simulink model "buck_boost_sim"  (R2020a)
settings: Solver=FixedStepAuto  StartTime=0.0  StopTime=sim_duration  FixedStep=1e-3  RelTol=1e-3
values from neighbouring files (symbols this model uses):
  A = double(eval(subs(A, u, ue)))    [linearizacija_simbolicki_script.m]    (also in linearizacija_simbolicki_skripta.m)
  B = double(eval(subs(B, [x1, x2], [x1e, x2e])))    [linearizacija_simbolicki_script.m]    (also in linearizacija_simbolicki_skripta.m)
  C = 470e-6    (= 0.00047)    [linearizacija_simbolicki_script.m]    (also in linearizacija_simbolicki_skripta.m)
  E = 12    [linearizacija_simbolicki_script.m]    (also in linearizacija_simbolicki_skripta.m)
  H = [0 1]    [linearizacija_simbolicki_script.m]    (also in linearizacija_simbolicki_skripta.m)
  L = 15.91e-3    (= 0.01591)    [linearizacija_simbolicki_script.m]    (also in linearizacija_simbolicki_skripta.m)
  R = 52    [linearizacija_simbolicki_script.m]    (also in linearizacija_simbolicki_skripta.m)
  sim_duration = 5    [projektovanje_kontrolera_script.m]
  ue = eval(ue)    [linearizacija_simbolicki_script.m]    (also in linearizacija_simbolicki_skripta.m)
  x2e = -22.5    [linearizacija_simbolicki_script.m]    (also in linearizacija_simbolicki_skripta.m)
undefined symbols (not defined in the file or in its folder): k_den, k_num
settings Model: Creator=HP  LastModifiedBy=HP

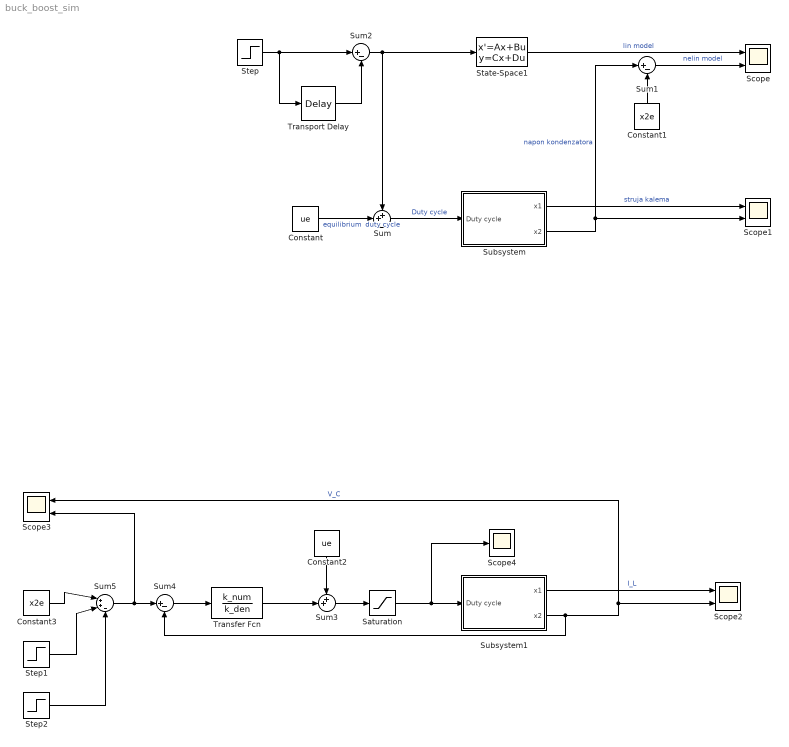
== system buck_boost_sim ==
  Constant : Constant  Value=ue
  Constant1 : Constant  Value=x2e
  Constant2 : Constant  Value=ue
  Constant3 : Constant  Value=x2e
  Saturation : Saturate  UpperLimit=1  LowerLimit=0
  Scope{,1..3} (4 alike) : Scope  NumInputPorts=2
  Scope4 : Scope
  State-Space1 : StateSpace  A=A  B=B  C=H  D=0  InitialCondition=0
  Step : Step  Time=0.3*sim_duration  After=0.03*ue  SampleTime=0
  Step1 : Step  Time=0.3*sim_duration  After=0.05 * x2e  SampleTime=0
  Step2 : Step  Time=0.4*sim_duration  After=0.1* x2e  SampleTime=0
  Subsystem : Subsystem
  Subsystem1 : Subsystem
  Sum : Sum  Inputs=++|
  Sum1 : Sum  Inputs=|+-
  Sum2 : Sum  Inputs=|+-
  Sum3 : Sum  Inputs=++|
  Sum4 : Sum  Inputs=|+-
  Sum5 : Sum  Inputs=|++-
  Transfer Fcn : TransferFcn  Numerator=k_num  Denominator=k_den
  Transport Delay : TransportDelay  DelayTime=0.1*sim_duration  BufferSize=2048
  wires:
  Subsystem/2(x2) -> Scope1/2, Sum1/1  "napon kondenzatora"
  Sum/1 -> Subsystem/1(Duty cycle)  "Duty cycle"
  Constant1/1 -> Sum1/2
  Sum1/1 -> Scope/2  "nelin model"
  State-Space1/1 -> Scope/1  "lin model"
  Constant/1 -> Sum/2  "equilibrium  duty cycle"
  Step/1 -> Transport Delay/1, Sum2/1
  Transport Delay/1 -> Sum2/2
  Sum2/1 -> State-Space1/1, Sum/1
  Subsystem/1(x1) -> Scope1/1  "struja kalema"
  Sum3/1 -> Saturation/1
  Constant2/1 -> Sum3/1
  Transfer Fcn/1 -> Sum3/2
  Sum4/1 -> Transfer Fcn/1
  Subsystem1/2(x2) -> Scope2/2, Scope3/1, Sum4/2  "V_C"
  Subsystem1/1(x1) -> Scope2/1  "I_L"
  Constant3/1 -> Sum5/1
  Sum5/1 -> Scope3/2, Sum4/1
  Step1/1 -> Sum5/2
  Step2/1 -> Sum5/3
  Saturation/1 -> Scope4/1, Subsystem1/1(Duty cycle)

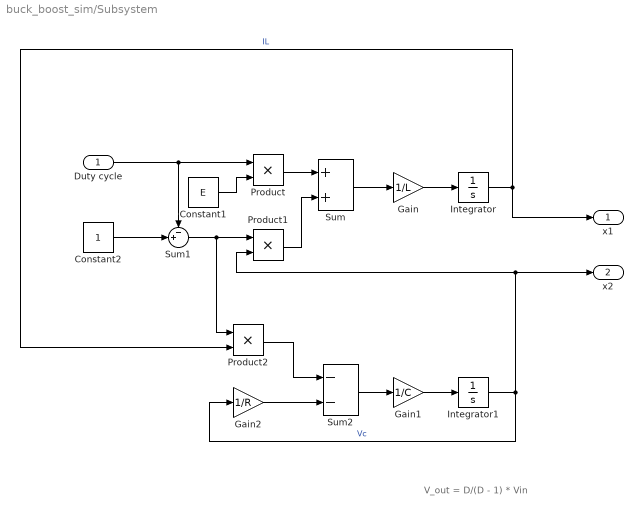
== system buck_boost_sim/Subsystem ==
  note: V_out = D/(D - 1) * Vin
  Duty cycle : Inport
  Constant1 : Constant  Value=E
  Constant2 : Constant
  Gain : Gain  Gain=1/L
  Gain1 : Gain  Gain=1/C
  Gain2 : Gain  Gain=1/R
  Integrator : Integrator
  Integrator1 : Integrator
  Product : Product
  Product1 : Product
  Product2 : Product
  Sum : Sum
  Sum1 : Sum  Inputs=-+|
  Sum2 : Sum  Inputs=--
  x1 : Outport
  x2 : Outport  Port=2
  wires:
  Product/1 -> Sum/1
  Product1/1 -> Sum/2
  Sum2/1 -> Gain1/1
  Constant1/1 -> Product/2
  Integrator1/1 -> Gain2/1, x2/1, Product1/2  "Vc"
  Gain1/1 -> Integrator1/1
  Constant2/1 -> Sum1/2
  Integrator/1 -> x1/1, Product2/2  "IL"
  Sum/1 -> Gain/1
  Gain2/1 -> Sum2/2
  Sum1/1 -> Product2/1, Product1/1
  Duty cycle/1 -> Sum1/1, Product/1
  Product2/1 -> Sum2/1
  Gain/1 -> Integrator/1

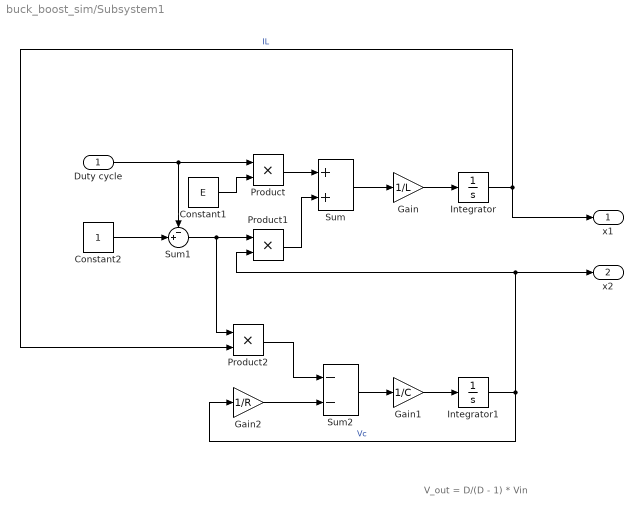
== system buck_boost_sim/Subsystem1 ==
  note: V_out = D/(D - 1) * Vin
  Duty cycle : Inport
  Constant1 : Constant  Value=E
  Constant2 : Constant
  Gain : Gain  Gain=1/L
  Gain1 : Gain  Gain=1/C
  Gain2 : Gain  Gain=1/R
  Integrator : Integrator
  Integrator1 : Integrator
  Product : Product
  Product1 : Product
  Product2 : Product
  Sum : Sum
  Sum1 : Sum  Inputs=-+|
  Sum2 : Sum  Inputs=--
  x1 : Outport
  x2 : Outport  Port=2
  wires:
  Product/1 -> Sum/1
  Product1/1 -> Sum/2
  Sum2/1 -> Gain1/1
  Constant1/1 -> Product/2
  Integrator1/1 -> Gain2/1, x2/1, Product1/2  "Vc"
  Gain1/1 -> Integrator1/1
  Constant2/1 -> Sum1/2
  Integrator/1 -> x1/1, Product2/2  "IL"
  Sum/1 -> Gain/1
  Gain2/1 -> Sum2/2
  Sum1/1 -> Product2/1, Product1/1
  Duty cycle/1 -> Sum1/1, Product/1
  Product2/1 -> Sum2/1
  Gain/1 -> Integrator/1
